simulink model "Subsystem1"  (R2020b)
settings: Solver=FixedStepAuto  StartTime=0.0  StopTime=10.0  FixedStep=0.2  RelTol=1e-3
settings Model: Creator=Pavan  LastModifiedBy=Pavan
settings DataIOCC: SaveOutput=off  SaveTime=off

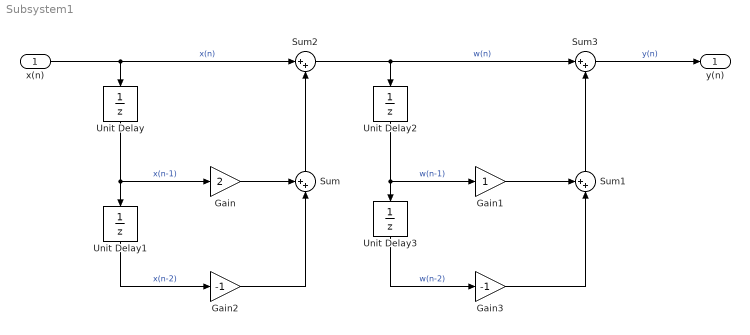
== system Subsystem1 ==
  x(n) : Inport  OutDataTypeStr=double  PortDimensions=1  SampleTime=[0.20000000000000001,0]
  Gain : Gain  Gain=2
  Gain1 : Gain
  Gain2 : Gain  Gain=-1
  Gain3 : Gain  Gain=-1
  Sum : Sum  Inputs=++|
  Sum1 : Sum  Inputs=++|
  Sum2 : Sum  Inputs=|++
  Sum3 : Sum  Inputs=|++
  Unit Delay{,1..3} (4 alike) : UnitDelay  SampleTime=-1  HasFrameUpgradeWarning=on
  y(n) : Outport  OutDataTypeStr=double  PortDimensions=1  SampleTime=[0.20000000000000001,0]
  wires:
  Sum1/1 -> Sum3/2
  Sum2/1 -> Unit Delay2/1, Sum3/1  "w(n)"
  x(n)/1 -> Unit Delay/1, Sum2/1  "x(n)"
  Unit Delay/1 -> Unit Delay1/1, Gain/1  "x(n-1)"
  Sum/1 -> Sum2/2
  Gain2/1 -> Sum/2
  Gain3/1 -> Sum1/2
  Unit Delay1/1 -> Gain2/1  "x(n-2)"
  Gain1/1 -> Sum1/1
  Unit Delay2/1 -> Unit Delay3/1, Gain1/1  "w(n-1)"
  Unit Delay3/1 -> Gain3/1  "w(n-2)"
  Gain/1 -> Sum/1
  Sum3/1 -> y(n)/1  "y(n)"
